simulink model "Vehicle_Model"  (R2022b)
settings: Solver=VariableStepAuto  StartTime=0.0  StopTime=10.0  RelTol=1e-3
libraries: matrix_library x1, vrlib x1
settings Model: Creator=alphabet1671  LastModifiedBy=Louis
settings OptimizationCC: ReuseModelBlockBuffer=on
settings RTWCC: GPUComputeCapability=5.0

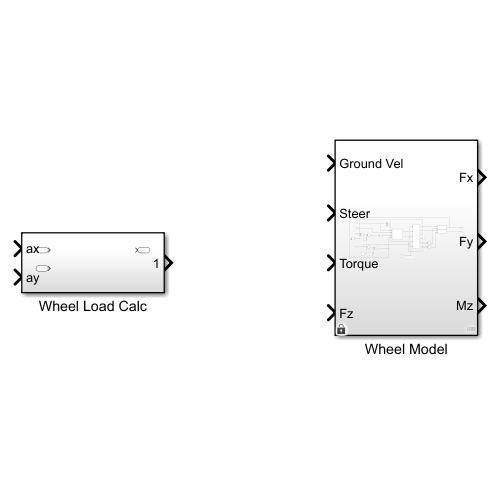
[thumbnail: Simulink's stored preview of the top-level diagram]
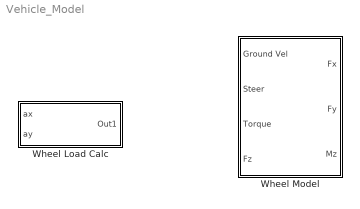
== system Vehicle_Model ==
  Wheel Load Calc : Subsystem
  Wheel Model : Subsystem

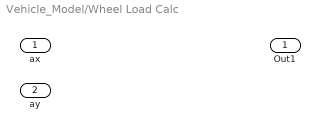
== system Vehicle_Model/Wheel Load Calc ==
  ax : Inport
  ay : Inport  Port=2
  Out1 : Outport

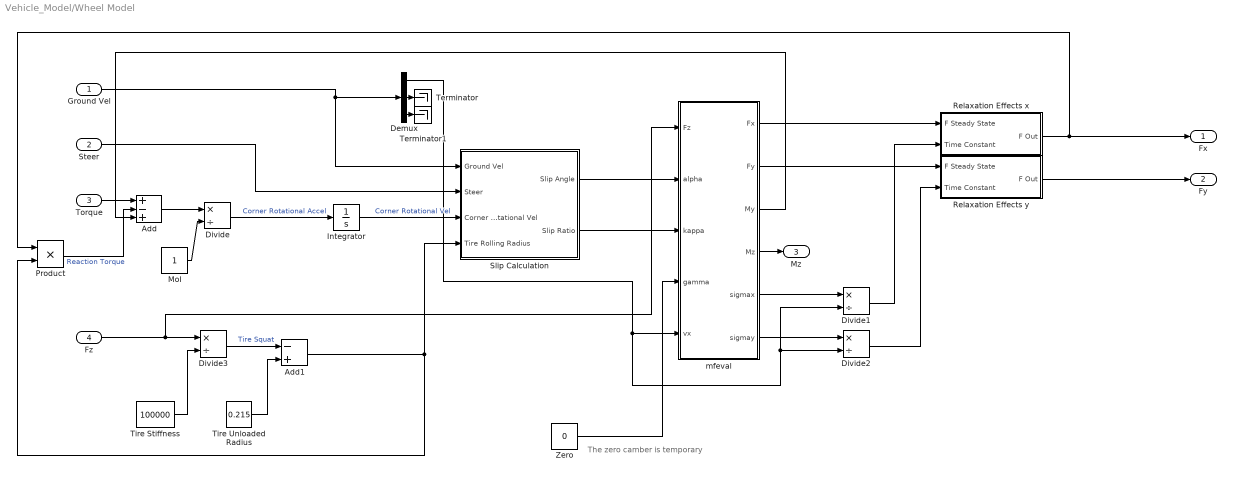
== system Vehicle_Model/Wheel Model ==
  note: The zero camber is temporary
  Ground Vel : Inport
  Steer : Inport  Port=2
  Torque : Inport  Port=3
  Fz : Inport  Port=4
  Add : Sum  Inputs=+-+
  Add1 : Sum  Inputs=-+
  Demux : Demux  Outputs=3
  Divide{,1..3} (4 alike) : Product  Inputs=*/
  Integrator : Integrator
  MoI : Constant
  Product : Product
  Relaxation Effects x : Subsystem
  Relaxation Effects y : Subsystem
  Slip Calculation : Subsystem
  Terminator : Terminator
  Terminator1 : Terminator
  Tire Stiffness : Constant  Value=100000
  Tire Unloaded Radius : Constant  Value=0.215
  Zero : Constant  Value=0  OutDataTypeStr=Inherit: Inherit via back propagation
  mfeval : MATLAB Function  TreatAsAtomicUnit=on
  Fx : Outport
  Fy : Outport  Port=2
  Mz : Outport  Port=3
  wires:
  Zero/1 -> mfeval/4(gamma)
  Tire Unloaded Radius/1 -> Add1/2
  Divide3/1 -> Add1/1  "Tire Squat"
  Tire Stiffness/1 -> Divide3/2
  Torque/1 -> Add/1
  MoI/1 -> Divide/2
  Divide/1 -> Integrator/1  "Corner Rotational Accel"
  Ground Vel/1 -> Demux/1, Slip Calculation/1(Ground Vel)
  Integrator/1 -> Slip Calculation/3(Corner Rotational Vel)  "Corner Rotational Vel"
  Steer/1 -> Slip Calculation/2(Steer)
  Slip Calculation/1(Slip Angle) -> mfeval/2(alpha)
  Slip Calculation/2(Slip Ratio) -> mfeval/3(kappa)
  Fz/1 -> mfeval/1(Fz), Divide3/1
  Add/1 -> Divide/1
  Add1/1 -> Product/2, Slip Calculation/4(Tire Rolling Radius)
  Product/1 -> Add/2  "Reaction Torque"
  mfeval/1(Fx) -> Relaxation Effects x/1(F Steady State)
  mfeval/2(Fy) -> Relaxation Effects y/1(F Steady State)
  mfeval/4(Mz) -> Mz/1
  Demux/1 -> mfeval/5(vx), Divide1/2, Divide2/2
  Demux/2 -> Terminator/1
  Demux/3 -> Terminator1/1
  mfeval/3(My) -> Add/3
  mfeval/5(sigmax) -> Divide1/1
  mfeval/6(sigmay) -> Divide2/1
  Divide1/1 -> Relaxation Effects x/2(Time Constant)
  Divide2/1 -> Relaxation Effects y/2(Time Constant)
  Relaxation Effects x/1(F Out) -> Fx/1, Product/1
  Relaxation Effects y/1(F Out) -> Fy/1

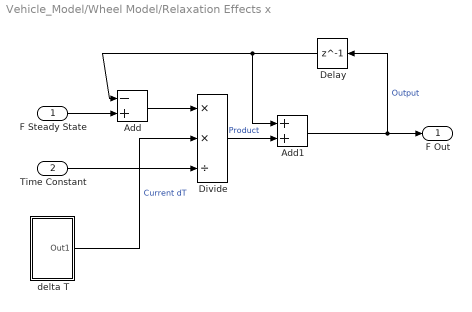
== system Vehicle_Model/Wheel Model/Relaxation Effects x ==
  F Steady State : Inport
  Time Constant : Inport  Port=2
  Add : Sum  Inputs=-+
  Add1 : Sum
  Delay : Delay  DelayLength=1  InitialCondition=0
  Divide : Product  Inputs=**/
  delta T : Subsystem
  F Out : Outport
  wires:
  F Steady State/1 -> Add/2
  Add/1 -> Divide/1
  Time Constant/1 -> Divide/3
  Add1/1 -> Delay/1, F Out/1  "Output"
  Delay/1 -> Add1/1, Add/1
  delta T/1(Out1) -> Divide/2  "Current dT"
  Divide/1 -> Add1/2  "Product"

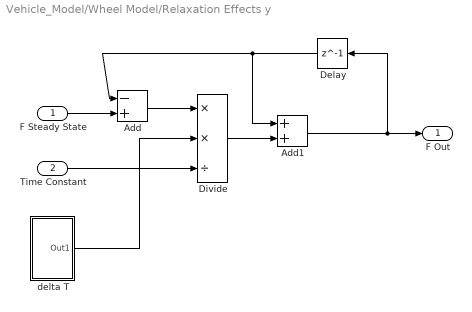
== system Vehicle_Model/Wheel Model/Relaxation Effects y ==
  F Steady State : Inport
  Time Constant : Inport  Port=2
  Add : Sum  Inputs=-+
  Add1 : Sum
  Delay : Delay  DelayLength=1  InitialCondition=0
  Divide : Product  Inputs=**/
  delta T : Subsystem
  F Out : Outport
  wires:
  F Steady State/1 -> Add/2
  Add/1 -> Divide/1
  Time Constant/1 -> Divide/3
  Add1/1 -> Delay/1, F Out/1
  Delay/1 -> Add1/1, Add/1
  delta T/1(Out1) -> Divide/2
  Divide/1 -> Add1/2

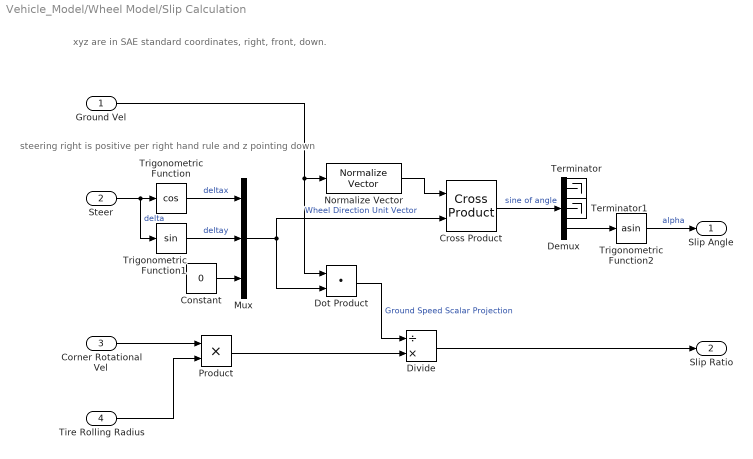
== system Vehicle_Model/Wheel Model/Slip Calculation ==
  note: steering right is positive per right hand rule and z pointing down
  note: xyz are in SAE standard coordinates, right, front, down.
  Ground Vel : Inport
  Steer : Inport  Port=2
  Corner Rotational Vel : Inport  Port=3
  Tire Rolling Radius : Inport  Port=4
  Constant : Constant  Value=0
  Cross Product : matrix_library/Cross Product
  Demux : Demux  Outputs=3
  Divide : Product  Inputs=/*
  Dot Product : DotProduct  OutDataTypeStr=double
  Mux : Mux  Inputs=3
  Normalize Vector : vrlib/Utilities/Normalize Vector  maxzero=0
  Product : Product
  Terminator : Terminator
  Terminator1 : Terminator
  Trigonometric Function : Trigonometry  Operator=cos
  Trigonometric Function1 : Trigonometry
  Trigonometric Function2 : Trigonometry  Operator=asin
  Slip Angle : Outport
  Slip Ratio : Outport  Port=2
  wires:
  Demux/3 -> Trigonometric Function2/1
  Constant/1 -> Mux/3
  Ground Vel/1 -> Dot Product/1, Normalize Vector/1
  Steer/1 -> Trigonometric Function1/1, Trigonometric Function/1  "delta"
  Corner Rotational Vel/1 -> Product/1
  Tire Rolling Radius/1 -> Product/2
  Product/1 -> Divide/2
  Trigonometric Function/1 -> Mux/1  "deltax"
  Trigonometric Function1/1 -> Mux/2  "deltay"
  Mux/1 -> Dot Product/2, Cross Product/2  "Wheel Direction Unit Vector"
  Cross Product/1 -> Demux/1  "sine of angle"
  Trigonometric Function2/1 -> Slip Angle/1  "alpha"
  Normalize Vector/1 -> Cross Product/1
  Dot Product/1 -> Divide/1  "Ground Speed Scalar Projection"
  Divide/1 -> Slip Ratio/1

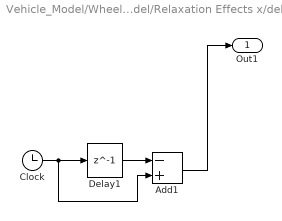
== system Vehicle_Model/Wheel Model/Relaxation Effects x/delta T ==
  Add1 : Sum  Inputs=-+
  Clock : Clock
  Delay1 : Delay  DelayLength=1  InitialCondition=0
  Out1 : Outport
  wires:
  Clock/1 -> Add1/2, Delay1/1
  Delay1/1 -> Add1/1
  Add1/1 -> Out1/1

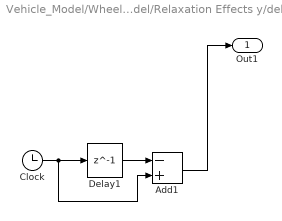
== system Vehicle_Model/Wheel Model/Relaxation Effects y/delta T ==
  Add1 : Sum  Inputs=-+
  Clock : Clock
  Delay1 : Delay  DelayLength=1  InitialCondition=0
  Out1 : Outport
  wires:
  Clock/1 -> Add1/2, Delay1/1
  Delay1/1 -> Add1/1
  Add1/1 -> Out1/1

== matlab function Vehicle_Model/Wheel Model/mfeval ==
  data: Fx output; Fy output; My output; Fz input; alpha input; kappa input; gamma input; vx input; Mz output; sigmax output; sigmay output
function [Fx, Fy, My, Mz, sigmax, sigmay]= runTireModel(Fz, alpha, kappa, gamma, vx)
coder.extrinsic('RunMFEval');
Fx = 0.0; Fy = 0.0; My = 0.0; Mz = 0.0; sigmax = 0.0; sigmay = 0.0;
[Fx, Fy, My, Mz, sigmax, sigmay] = RunMFEval(Fz, alpha, kappa, gamma, vx);
end
